simulink model "Task_1B"  (R2022a)
settings: Solver=VariableStepAuto  StartTime=0.0  StopTime=10.0  RelTol=1e-3
values from neighbouring files (symbols this model uses):
  d_COM = R_robot * cos(theta_wheels)    [Parameter_Setup.m]
  J_total = J_robot + (m_total * (d_COM^2))    [Parameter_Setup.m]
  L_wheel = R_robot * sin(theta_wheels)    [Parameter_Setup.m]
  m_total = m_load + m_robot    (= 40)    [Parameter_Setup.m]
  R_wheel = D_wheel/2    (= 0.05)    [Parameter_Setup.m]
settings Model: Creator=jpcas  LastModifiedBy=jpcas

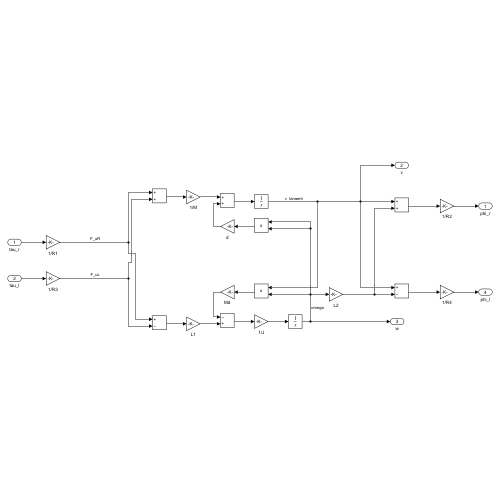
[thumbnail: Simulink's stored preview of the top-level diagram]
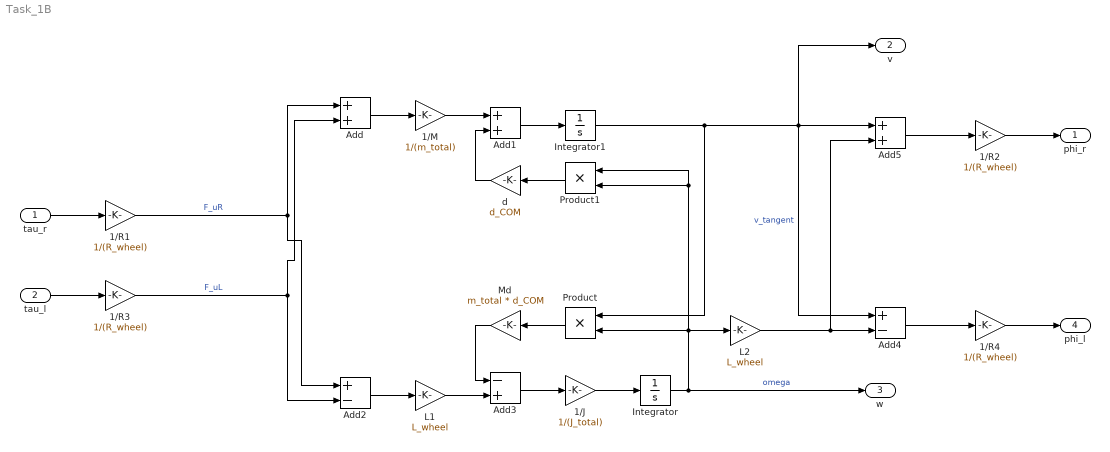
== system Task_1B ==
  tau_r : Inport
  tau_l : Inport  Port=2
  1/J : Gain  Gain=1/(J_total)
  1/M : Gain  Gain=1/(m_total)
  1/R{1..4} (4 alike) : Gain  Gain=1/(R_wheel)
  Add : Sum
  Add1 : Sum
  Add2 : Sum  Inputs=+-
  Add3 : Sum  Inputs=-+
  Add4 : Sum  Inputs=+-
  Add5 : Sum
  Integrator : Integrator
  Integrator1 : Integrator
  L1 : Gain  Gain=L_wheel
  L2 : Gain  Gain=L_wheel
  Md : Gain  Gain=m_total * d_COM
  Product : Product
  Product1 : Product
  d : Gain  Gain=d_COM
  phi_r : Outport
  v : Outport  Port=2
  w : Outport  Port=3
  phi_l : Outport  Port=4
  wires:
  1/R1/1 -> Add2/1, Add/1  "F_uR"
  Add/1 -> 1/M/1
  1/R3/1 -> Add/2, Add2/2  "F_uL"
  Add2/1 -> L1/1
  1/M/1 -> Add1/1
  Md/1 -> Add3/1
  Product/1 -> Md/1
  L1/1 -> Add3/2
  Add3/1 -> 1/J/1
  1/J/1 -> Integrator/1
  d/1 -> Add1/2
  Integrator/1 -> w/1, Product1/1, Product1/2, L2/1, Product/2  "omega"
  Product1/1 -> d/1
  Integrator1/1 -> Product/1, v/1, Add4/1, Add5/1  "v_tangent"
  Add1/1 -> Integrator1/1
  L2/1 -> Add4/2, Add5/2
  tau_r/1 -> 1/R1/1
  1/R2/1 -> phi_r/1
  tau_l/1 -> 1/R3/1
  1/R4/1 -> phi_l/1
  Add4/1 -> 1/R4/1
  Add5/1 -> 1/R2/1
